simulink model "tail_chase"  (R2024b)
settings: Solver=ode4  StartTime=0.0  StopTime=tf  FixedStep=0.01  RelTol=1e-3
values from neighbouring files (symbols this model uses):
  e0 = lambda0*N - gamma0 - (N - 1)*gamma_T0    [parameters_new.m]
  gamma0 = deg2rad(90)    [parameters_new.m]
  Ki = (0.83/damping_ratio)^2    [parameters_new.m]
  Kp = 2*damping_ratio*sqrt(Ki)    [parameters_new.m]
  main_guidance = 1    [parameters_new.m]
  vP = 25    [parameters_new.m]
  x_switch = 200    [parameters_new.m]
  xP_initial = 0    [parameters_new.m]
  yP_initial = 0    [parameters_new.m]
undefined symbols (not defined in the file or in its folder): DiscIntNeverNeededParam
settings Model: Creator=AK127381  LastModifiedBy=AK127381
settings DebuggingCC: AlgebraicLoopMsg=none

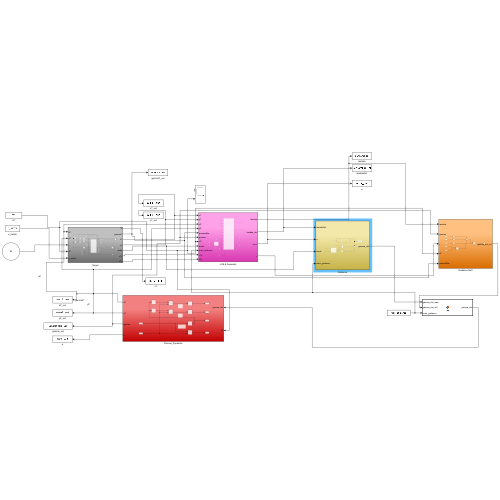
[thumbnail: Simulink's stored preview of the top-level diagram]
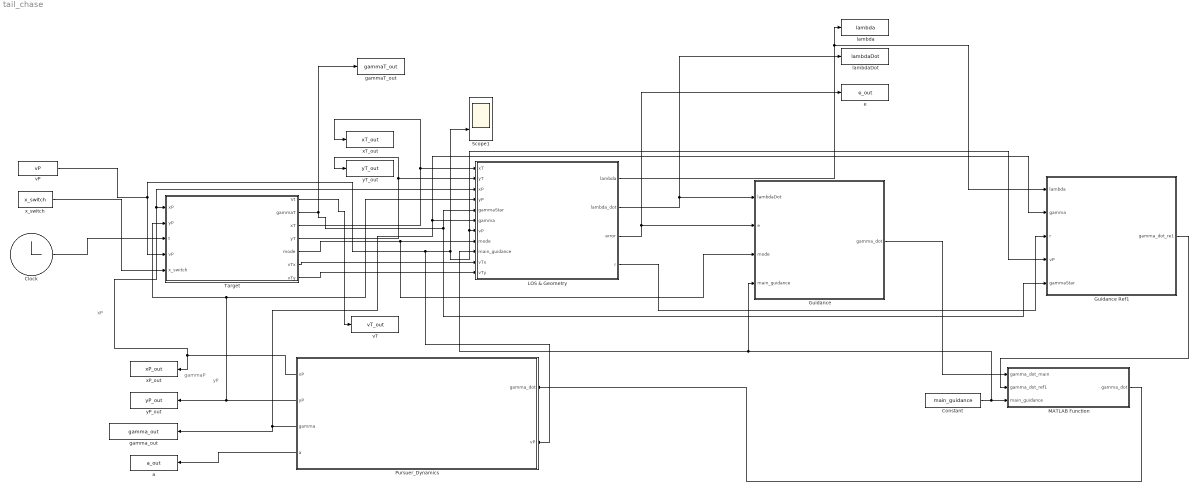
== system tail_chase ==
  note: yP
  note: gammaP
  note: xP
  Clock : Clock
      settings: Decimation=tf
  Constant : Constant  Value=main_guidance
  "Guidance " : Subsystem
  Guidance Ref1 : Subsystem
  LOS & Geometry : Subsystem
  MATLAB Function : MATLAB Function  TreatAsAtomicUnit=on
  Pursuer_Dynamics : Subsystem
  Scope1 : Scope  NumInputPorts=2
  Target : Subsystem
  a : ToWorkspace  VariableName=a_out  SampleTime=-1
      settings: Save2DSignal=2-D array (concatenate along first dimension)
  e : ToWorkspace  VariableName=e_out  SampleTime=-1
      settings: Save2DSignal=2-D array (concatenate along first dimension)
  gammaT_out : ToWorkspace  VariableName=gammaT_out  SampleTime=-1
      settings: Save2DSignal=2-D array (concatenate along first dimension)
  gamma_out : ToWorkspace  VariableName=gamma_out  SampleTime=-1
      settings: Save2DSignal=2-D array (concatenate along first dimension)
  lambda : ToWorkspace  VariableName=lambda  SampleTime=-1
      settings: Save2DSignal=2-D array (concatenate along first dimension)
  lambdaDot : ToWorkspace  VariableName=lambdaDot  SampleTime=-1
      settings: Save2DSignal=2-D array (concatenate along first dimension)
  vP : Constant  Value=vP
  vT : ToWorkspace  VariableName=vT_out  SampleTime=-1
      settings: Save2DSignal=2-D array (concatenate along first dimension)
  xP_out : ToWorkspace  VariableName=xP_out  SampleTime=-1
      settings: Save2DSignal=2-D array (concatenate along first dimension)
  xT_out : ToWorkspace  VariableName=xT_out  SampleTime=-1
      settings: Save2DSignal=2-D array (concatenate along first dimension)
  x_switch : Constant  Value=x_switch
  yP_out : ToWorkspace  VariableName=yP_out  SampleTime=-1
      settings: Save2DSignal=2-D array (concatenate along first dimension)
  yT_out : ToWorkspace  VariableName=yT_out  SampleTime=-1
      settings: Save2DSignal=2-D array (concatenate along first dimension)
  wires:
  Pursuer_Dynamics/4(a) -> a/1
  Pursuer_Dynamics/3(gamma) -> gamma_out/1, Guidance Ref1/2(gamma), LOS & Geometry/6(gamma)
  vP/1 -> Target/4(vP), Pursuer_Dynamics/2(vP), Guidance Ref1/4(vP), LOS & Geometry/7(vP), Scope1/2
  Clock/1 -> Target/3(t)
  LOS & Geometry/3(error) -> e/1, "Guidance "/2(e)
  Pursuer_Dynamics/2(yP) -> LOS & Geometry/4(yP), Target/2(yP), yP_out/1
  "Guidance "/1(gamma_dot) -> MATLAB Function/1(gamma_dot_main)
  Pursuer_Dynamics/1(xP) -> LOS & Geometry/3(xP), Target/1(xP), xP_out/1
  LOS & Geometry/1(lambda) -> lambda/1, Guidance Ref1/1(lambda)
  MATLAB Function/1(gamma_dot) -> Pursuer_Dynamics/1(gamma_dot)
  LOS & Geometry/2(lambda_dot) -> lambdaDot/1, "Guidance "/1(lambdaDot)
  Target/1(Vt) -> vT/1
  Target/3(xT) -> xT_out/1, LOS & Geometry/1(xT)
  Target/4(yT) -> yT_out/1, LOS & Geometry/2(yT)
  Target/2(gammaT) -> Guidance Ref1/5(gammaStar), LOS & Geometry/5(gammaStar), gammaT_out/1
  x_switch/1 -> Target/5(x_switch)
  LOS & Geometry/4(r) -> Guidance Ref1/3(r)
  Guidance Ref1/1(gamma_dot_re1) -> MATLAB Function/2(gamma_dot_ref1)
  Constant/1 -> "Guidance "/4(main_guidance), LOS & Geometry/9(main_guidance), MATLAB Function/3(main_guidance)
  Target/6(vTx) -> LOS & Geometry/10(vTx)
  Target/5(mode) -> LOS & Geometry/8(mode), "Guidance "/3(mode)
  Target/7(vTy) -> LOS & Geometry/11(vTy)

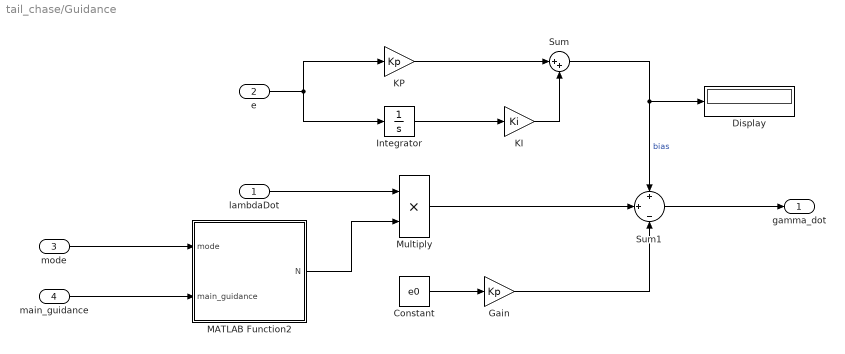
== system tail_chase/Guidance  ==
  lambdaDot : Inport
  e : Inport  Port=2
  mode : Inport  Port=3
  main_guidance : Inport  Port=4
  Constant : Constant  Value=e0
  Display : Display
  Gain : Gain  Gain=Kp
  Integrator : Integrator  InitialCondition=e0
  KI : Gain  Gain=Ki
  KP : Gain  Gain=Kp
  MATLAB Function2 : MATLAB Function  TreatAsAtomicUnit=on
  Multiply : Product
  Sum : Sum  Inputs=|++
  Sum1 : Sum  Inputs=+|+|-
  gamma_dot : Outport
  wires:
  e/1 -> KP/1, Integrator/1
  KP/1 -> Sum/1
  lambdaDot/1 -> Multiply/1
  Integrator/1 -> KI/1
  KI/1 -> Sum/2
  Sum/1 -> Display/1, Sum1/1  "bias"
  Sum1/1 -> gamma_dot/1
  Multiply/1 -> Sum1/2
  Constant/1 -> Gain/1
  Gain/1 -> Sum1/3
  main_guidance/1 -> MATLAB Function2/2(main_guidance)
  MATLAB Function2/1(N) -> Multiply/2
  mode/1 -> MATLAB Function2/1(mode)

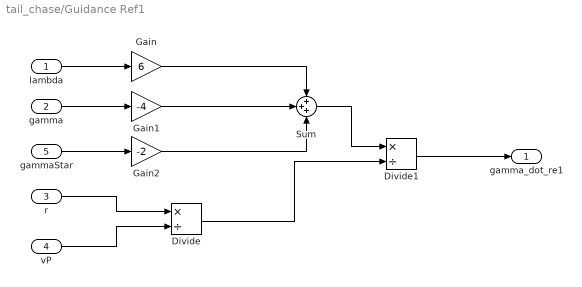
== system tail_chase/Guidance Ref1 ==
  lambda : Inport
  gamma : Inport  Port=2
  r : Inport  Port=3
  vP : Inport  Port=4
  gammaStar : Inport  Port=5
  Divide : Product  Inputs=*/
  Divide1 : Product  Inputs=*/
  Gain : Gain  Gain=6
  Gain1 : Gain  Gain=-4
  Gain2 : Gain  Gain=-2
  Sum : Sum  Inputs=+++
  gamma_dot_re1 : Outport
  wires:
  lambda/1 -> Gain/1
  gamma/1 -> Gain1/1
  gammaStar/1 -> Gain2/1
  Gain/1 -> Sum/1
  Gain1/1 -> Sum/2
  Gain2/1 -> Sum/3
  Sum/1 -> Divide1/1
  Divide/1 -> Divide1/2
  r/1 -> Divide/1
  vP/1 -> Divide/2
  Divide1/1 -> gamma_dot_re1/1

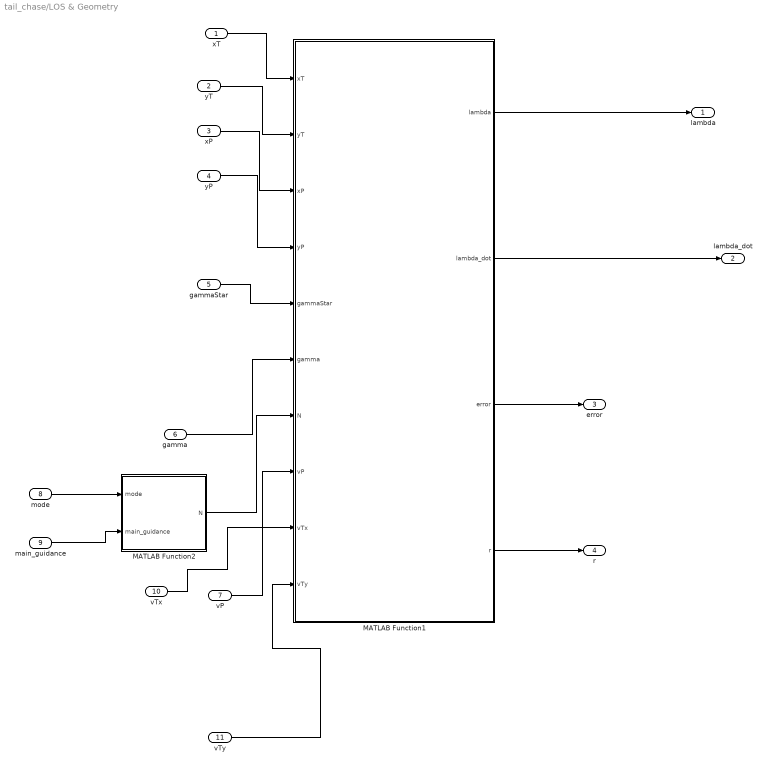
== system tail_chase/LOS & Geometry ==
  xT : Inport
  yT : Inport  Port=2
  xP : Inport  Port=3
  yP : Inport  Port=4
  gammaStar : Inport  Port=5
  gamma : Inport  Port=6
  vP : Inport  Port=7
  mode : Inport  Port=8
  main_guidance : Inport  Port=9
  vTx : Inport  Port=10
  vTy : Inport  Port=11
  MATLAB Function1 : MATLAB Function  TreatAsAtomicUnit=on
  MATLAB Function2 : MATLAB Function  TreatAsAtomicUnit=on
  lambda : Outport
  lambda_dot : Outport  Port=2
  error : Outport  Port=3
  r : Outport  Port=4
  wires:
  xT/1 -> MATLAB Function1/1(xT)
  yT/1 -> MATLAB Function1/2(yT)
  xP/1 -> MATLAB Function1/3(xP)
  yP/1 -> MATLAB Function1/4(yP)
  gammaStar/1 -> MATLAB Function1/5(gammaStar)
  MATLAB Function1/3(error) -> error/1
  gamma/1 -> MATLAB Function1/6(gamma)
  MATLAB Function2/1(N) -> MATLAB Function1/7(N)
  MATLAB Function1/1(lambda) -> lambda/1
  vP/1 -> MATLAB Function1/8(vP)
  mode/1 -> MATLAB Function2/1(mode)
  MATLAB Function1/4(r) -> r/1
  main_guidance/1 -> MATLAB Function2/2(main_guidance)
  MATLAB Function1/2(lambda_dot) -> lambda_dot/1
  vTx/1 -> MATLAB Function1/9(vTx)
  vTy/1 -> MATLAB Function1/10(vTy)

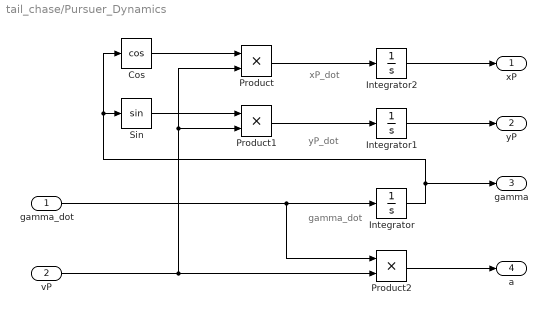
== system tail_chase/Pursuer_Dynamics ==
  note: gamma_dot
  note: xP_dot
  note: yP_dot
  gamma_dot : Inport
  vP : Inport  Port=2
  Cos : Trigonometry  Operator=cos
  Integrator : Integrator  InitialCondition=gamma0
  Integrator1 : Integrator  InitialCondition=yP_initial
  Integrator2 : Integrator  InitialCondition=xP_initial
  Product : Product
  Product1 : Product
  Product2 : Product
  Sin : Trigonometry
  xP : Outport
  yP : Outport  Port=2
  gamma : Outport  Port=3
  a : Outport  Port=4
  wires:
  vP/1 -> Product/2, Product1/2, Product2/2
  gamma_dot/1 -> Integrator/1, Product2/1
  Integrator/1 -> Cos/1, Sin/1, gamma/1
  Integrator2/1 -> xP/1
  Product/1 -> Integrator2/1
  Cos/1 -> Product/1
  Sin/1 -> Product1/1
  Product1/1 -> Integrator1/1
  Integrator1/1 -> yP/1
  Product2/1 -> a/1

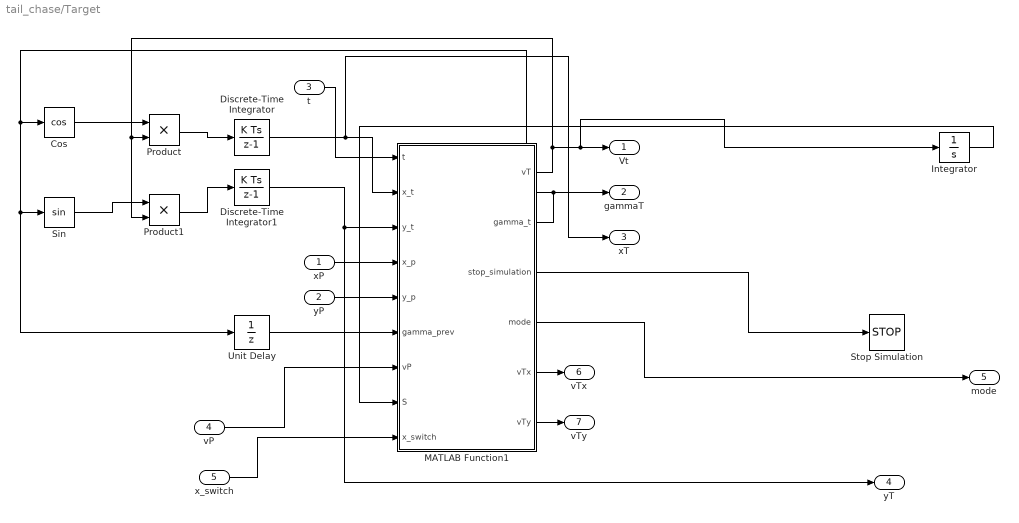
== system tail_chase/Target ==
  xP : Inport
  yP : Inport  Port=2
  t : Inport  Port=3
  vP : Inport  Port=4
  x_switch : Inport  Port=5
  Cos : Trigonometry  Operator=cos
  Discrete-Time Integrator : DiscreteIntegrator  SampleTime=0.01  ICPrevOutput=DiscIntNeverNeededParam  ICPrevScaledInput=DiscIntNeverNeededParam
  Discrete-Time Integrator1 : DiscreteIntegrator  InitialCondition=100  SampleTime=0.01  ICPrevOutput=DiscIntNeverNeededParam  ICPrevScaledInput=DiscIntNeverNeededParam
  Integrator : Integrator
  MATLAB Function1 : MATLAB Function  TreatAsAtomicUnit=on
  Product : Product
  Product1 : Product
  Sin : Trigonometry
  Stop Simulation : Stop
  Unit Delay : UnitDelay  SampleTime=0.01  HasFrameUpgradeWarning=on
  Vt : Outport
  gammaT : Outport  Port=2
  xT : Outport  Port=3
  yT : Outport  Port=4
  mode : Outport  Port=5
  vTx : Outport  Port=6
  vTy : Outport  Port=7
  wires:
  Sin/1 -> Product1/1
  MATLAB Function1/2(gamma_t) -> Unit Delay/1, Sin/1, Cos/1, gammaT/1
  Discrete-Time Integrator1/1 -> yT/1, MATLAB Function1/3(y_t)
  Unit Delay/1 -> MATLAB Function1/6(gamma_prev)
  Product1/1 -> Discrete-Time Integrator1/1
  t/1 -> MATLAB Function1/1(t)
  Product/1 -> Discrete-Time Integrator/1
  xP/1 -> MATLAB Function1/4(x_p)
  Cos/1 -> Product/1
  yP/1 -> MATLAB Function1/5(y_p)
  MATLAB Function1/1(vT) -> Product1/2, Product/2, Integrator/1, Vt/1
  vP/1 -> MATLAB Function1/7(vP)
  Discrete-Time Integrator/1 -> xT/1, MATLAB Function1/2(x_t)
  MATLAB Function1/3(stop_simulation) -> Stop Simulation/1
  MATLAB Function1/4(mode) -> mode/1
  Integrator/1 -> MATLAB Function1/8(S)
  x_switch/1 -> MATLAB Function1/9(x_switch)
  MATLAB Function1/6(vTy) -> vTy/1
  MATLAB Function1/5(vTx) -> vTx/1

== matlab function tail_chase/Guidance /MATLAB Function2 ==
  data: mode input; N output; main_guidance input
function N = fcn(mode, main_guidance)

    if main_guidance == 0
        N=3
    else
        if mode == 1
            N = 2
        else
            N = 1.25
        end
    end
end

== matlab function tail_chase/LOS & Geometry/MATLAB Function1 ==
  data: lambda output; xT input; yT input; xP input; yP input; gammaStar input; lambda_dot output; error output; gamma input; N input; vP input; r output; vTx input; vTy input
function [ lambda,  lambda_dot, error, r] = ref9(xT, yT, xP, yP, gammaStar, gamma, N, vP, vTx, vTy)
    

    %% 1) Relative position 
    dx = xT - xP;
    dy = yT - yP;

    r = hypot(dx, dy);
    %% 2) LOS angle 
    lambda = atan2(dy, dx); 
    % force into [0,2*pi)
    lambda = mod(lambda, 2*pi);

    % 5) Pursuer Velecities
    vPx = cos(gamma)*vP;
    vPy = sin(gamma)*vP;

    % lambda_dot = vT*sin(gammaStar - lambda)/r;   % ref 9
    
    % lambda_dot = -(dx*vy - dy*vx)/(r*r);

    %  Relative Velocities
    dvx = vTx - vPx;
    dvy = vTy - vPy;

    % 8) LOS rate
    lambda_dot = (dx*dvy - dy*dvx)/(r*r);
    
    error = N*lambda - gamma - (N-1)*gammaStar;  % N is fixed

== matlab function tail_chase/LOS & Geometry/MATLAB Function2 ==
  data: mode input; N output; main_guidance input
function N = fcn(mode, main_guidance)

    if main_guidance == 0
        N=3
    else
        if mode == 1
            N = 2
        else
            N = 1.25
        end
    end
end

== matlab function tail_chase/MATLAB Function ==
  data: gamma_dot_main input; gamma_dot output; gamma_dot_ref1 input; main_guidance input
function gamma_dot = fcn(gamma_dot_main, gamma_dot_ref1, main_guidance)
    
    if main_guidance== 0
        gamma_dot = gamma_dot_ref1;
        disp('Reference 1 guidance law is engaged')
    else 
        gamma_dot = gamma_dot_main;
        disp( 'main guidance law is engaged')
    end
end

== matlab function tail_chase/Target/MATLAB Function1 ==
  data: t input; x_t input; y_t input; x_p input; vT output; y_p input; gamma_prev input; gamma_t output; vP input; stop_simulation output; S input; mode output; x_switch input; vTx output; vTy output
function [vT, gamma_t, stop_simulation, mode, vTx, vTy] = targetLogic(t, x_t, y_t, ...
                                      x_p, y_p, gamma_prev, vP, S, x_switch)
    % --- range to pursuer
    r = hypot(x_t - x_p, y_t - y_p);
    
    % --- speed profile
    vT = 25 * (vP / r);            % Eq.  given by OP
    stop_simulation =0
    if S >=x_switch
        t
        mode = 1 %curved
        W_k      = vT / 100;      % instantaneous angular-rate
        gamma_t  = gamma_prev + W_k * 0.01
        
        if gamma_t >= 2*pi
            stop_simulation = 1
        else 
            stop_simulation = 0
        end
    else
        gamma_t = 0;
        mode = 0  %linear
    end

    vTx = cos(gamma_t)*vT;
    vTy = sin(gamma_t)*vT;

end
